simulink model "parabolic_system"  (R2024b)
settings: Solver=VariableStepAuto  StartTime=0.0  StopTime=inf  RelTol=1e-3
values from neighbouring files (symbols this model uses):
  A = 0.049    [for_the_parameters.m]
  cW = 0.35    [for_the_parameters.m]
  g = 9.81    [for_the_parameters.m]
  m = 0.5    [for_the_parameters.m]
  phi_0 = pi/4    (= 0.785398163397)    [for_the_parameters.m]
  rho = 1.25    [for_the_parameters.m]
  y_h0 = 0    [for_the_parameters.m]
  y_v0 = 0    [for_the_parameters.m]
settings Model: Creator=kavin  LastModifiedBy=kavin

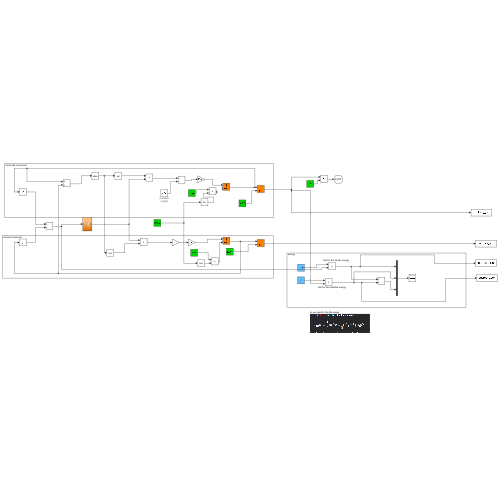
[thumbnail: Simulink's stored preview of the top-level diagram]
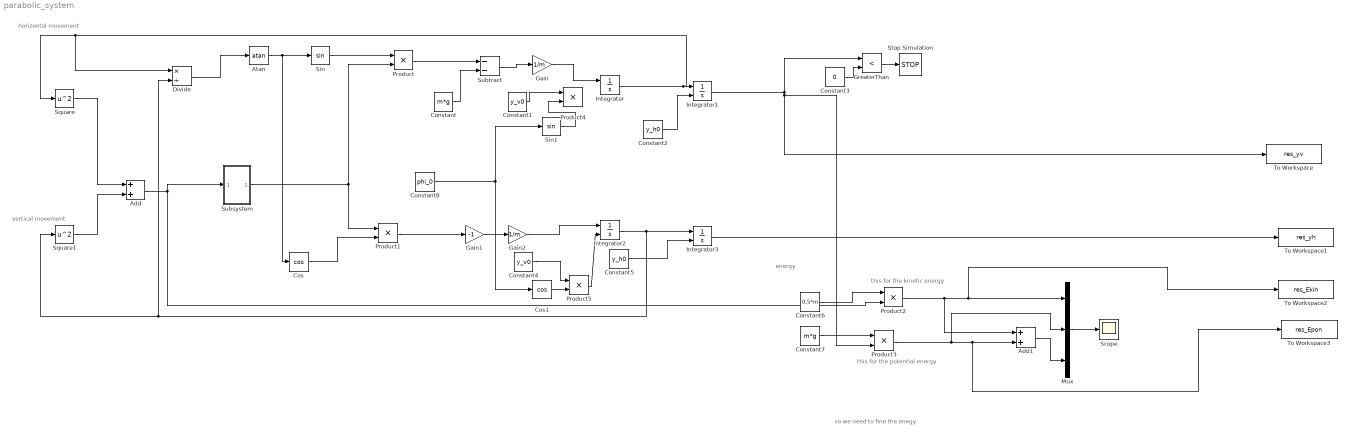
== system parabolic_system ==
  note: this for the potential energy
  note: this for the kinetic energy
  note: so we need to fine the enegy
  note: vertical movement
  note: horizontal movement
  note: energy
  Add : Sum
  Add1 : Sum
  Atan : Trigonometry  Operator=atan
  Constant : Constant  Value=m*g
      settings: AttributesFormatString=|
      | %<BlockType>
      | m*g(N)
  Constant1 : Constant  Value=y_v0
  Constant2 : Constant  Value=y_h0
  Constant3 : Constant  Value=0
  Constant4 : Constant  Value=y_v0
  Constant5 : Constant  Value=y_h0
  Constant6 : Constant  Value=0.5*m
  Constant7 : Constant  Value=m*g
  Constant8 : Constant  Value=phi_0
  Cos : Trigonometry  Operator=cos
  Cos1 : Trigonometry  Operator=cos
  Divide : Product  Inputs=*/
  Gain : Gain  Gain=1/m
  Gain1 : Gain  Gain=-1
  Gain2 : Gain  Gain=1/m
  GreaterThan : RelationalOperator  Operator=<  OutDataTypeStr=boolean  RndMeth=Simplest  InputSameDT=off
  Integrator{,1..3} (4 alike) : Integrator  InitialConditionSource=external
  Mux : Mux  Inputs=3
  Product{,1..5} (6 alike) : Product
  Scope : Scope
  Sin : Trigonometry
  Sin1 : Trigonometry
  Square : Math  Operator=square
  Square1 : Math  Operator=square
  Stop Simulation : Stop
  Subsystem : Subsystem
  Subtract : Sum  Inputs=--
  To Workspace : ToWorkspace  VariableName=res_yv  SaveFormat=Timeseries  SampleTime=-1
  To Workspace1 : ToWorkspace  VariableName=res_yh  SaveFormat=Timeseries  SampleTime=-1
  To Workspace2 : ToWorkspace  VariableName=res_Ekin  SaveFormat=Timeseries  SampleTime=-1
  To Workspace3 : ToWorkspace  VariableName=res_Epon  SaveFormat=Timeseries  SampleTime=-1
  wires:
  Add/1 -> Subsystem/1(In1), Product2/2
  Square/1 -> Add/1
  Integrator/1 -> Square/1, Divide/1, Integrator1/1
  Divide/1 -> Atan/1
  Atan/1 -> Cos/1, Sin/1
  Sin/1 -> Product/1
  Subsystem/1(Out1) -> Product/2, Product1/1
  Product/1 -> Subtract/1
  Constant/1 -> Subtract/2
  Subtract/1 -> Gain/1
  Gain/1 -> Integrator/1
  Constant1/1 -> Product4/1
  Constant2/1 -> Integrator1/2
  Constant3/1 -> GreaterThan/2
  GreaterThan/1 -> Stop Simulation/1
  Integrator1/1 -> Product3/2, To Workspace/1, GreaterThan/1
  Square1/1 -> Add/2
  Integrator2/1 -> Square1/1, Divide/2, Integrator3/1
  Cos/1 -> Product1/2
  Gain1/1 -> Gain2/1
  Product1/1 -> Gain1/1
  Gain2/1 -> Integrator2/1
  Constant4/1 -> Product5/1
  Constant5/1 -> Integrator3/2
  Integrator3/1 -> To Workspace1/1
  Product3/1 -> To Workspace3/1, Add1/2, Mux/2
  Product2/1 -> Add1/1, To Workspace2/1, Mux/1
  Add1/1 -> Mux/3
  Constant6/1 -> Product2/1
  Constant7/1 -> Product3/1
  Mux/1 -> Scope/1
  Sin1/1 -> Product4/2
  Constant8/1 -> Cos1/1, Sin1/1
  Product5/1 -> Integrator2/2
  Cos1/1 -> Product5/2

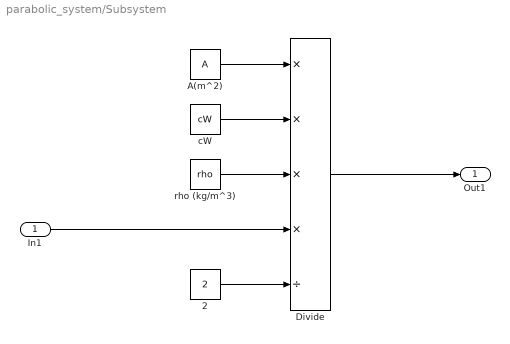
== system parabolic_system/Subsystem ==
  In1 : Inport
  2 : Constant  Value=2
  A(m^2) : Constant  Value=A
  Divide : Product  Inputs=****/
  cW : Constant  Value=cW
  rho (kg/m^3) : Constant  Value=rho
  Out1 : Outport
  wires:
  A(m^2)/1 -> Divide/1
  rho (kg/m^3)/1 -> Divide/3
  cW/1 -> Divide/2
  2/1 -> Divide/5
  Divide/1 -> Out1/1
  In1/1 -> Divide/4
